simulink model "sampleModel1691"  (R2023a)
settings: Solver=VariableStepAuto  StartTime=0.0  StopTime=10.0  RelTol=1e-3
libraries: hdlsllib x5
settings Model: Creator=user1  LastModifiedBy=user1

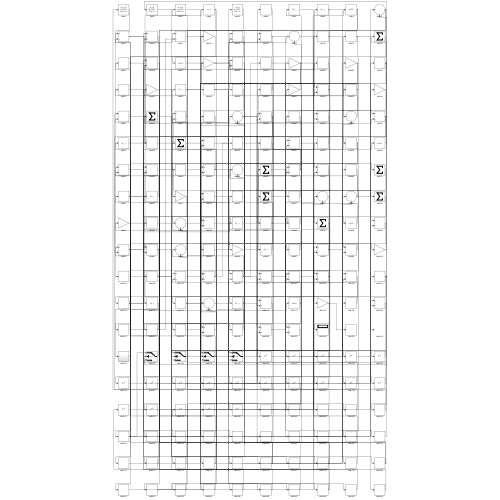
[thumbnail: Simulink's stored preview of the top-level diagram]
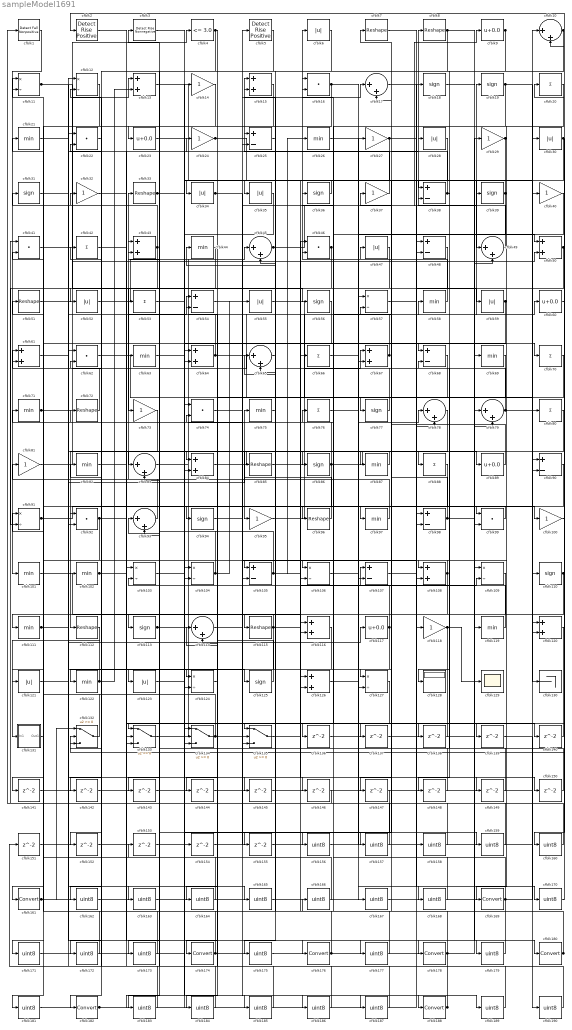
== system sampleModel1691 ==
  cfblk1 : hdlsllib/Logic and Bit Operations/Detect Fall Nonpositive  vinit=0  OutDataTypeStr=boolean
  cfblk{10,17,45,49,65,78..79,83,93,114} (10 alike) : Sum  Inputs=|++
  cfblk{14,24,27,29,32,37,40,73,81,95,100,118} (12 alike) : Gain
  cfblk{21,26,44,58,63,69,71,75,82,87,97,101..102,111,119,122} (16 alike) : MinMax
  cfblk{11..12,57,91,103..104,106,109,124,127} (10 alike) : Product  Inputs=*/  RndMeth=Zero  SaturateOnIntegerOverflow=on
  cfblk{25,38,48,54,68,90,98,105,107} (9 alike) : Sum  Inputs=+-
  cfblk{13,15,43,50,61,64,67,84,108,116,120,126} (12 alike) : Sum
  cfblk{18..19,31,36,39,56,77,86,94,110,113,125} (12 alike) : Signum
  cfblk{7..8,33,51,72,85,96,112,115} (9 alike) : Reshape
  cfblk{9,23,60,89,117} (5 alike) : Bias  Bias=0.0  SaturateOnIntegerOverflow=off
  cfblk{6,28,30,34..35,47,52,55,59,121,123} (11 alike) : Abs  SaturateOnIntegerOverflow=off
  cfblk128 : Display
  cfblk129 : Scope
  cfblk130 : Terminator
  cfblk131 : Subsystem
      settings: LibrarySourceBlock=|
      | hdlsllib/Ports &
      | Subsystems/Subsystem
  cfblk{132..135} (4 alike) : Switch  SaturateOnIntegerOverflow=off  InputSameDT=off
  cfblk{136..155} (20 alike) : Delay  SampleTime=1
  cfblk{156..160,162..168,170..173,175,177,179,181,183..187,189..190} (27 alike) : DataTypeConversion  OutDataTypeStr=uint8  SaturateOnIntegerOverflow=off  RndMeth=Floor
  cfblk{16,22,41,46,62,74,92,99} (8 alike) : DotProduct  OutDataTypeStr=Inherit: Inherit via internal rule
  cfblk{161,169,174,176,178,180,182,188} (8 alike) : DataTypeConversion  SaturateOnIntegerOverflow=off  RndMeth=Floor
  cfblk2 : hdlsllib/Logic and Bit Operations/Detect Rise Positive  vinit=0  OutDataTypeStr=boolean
  cfblk{20,42,53,66,70,76,80,88} (8 alike) : Sum  Inputs=+
  cfblk3 : hdlsllib/Logic and Bit Operations/Detect Rise Nonnegative  vinit=0  OutDataTypeStr=boolean
  cfblk4 : hdlsllib/Logic and Bit Operations/Compare To Constant  relop=<=  const=3.0  OutDataTypeStr=boolean
  cfblk5 : hdlsllib/Logic and Bit Operations/Detect Rise Positive  vinit=0  OutDataTypeStr=boolean
  wires:
  cfblk37/1 -> cfblk15/1
  cfblk36/1 -> cfblk34/1
  cfblk1/1 -> cfblk101/1
  cfblk93/1 -> cfblk33/1
  cfblk133/1 -> cfblk60/1
  cfblk117/1 -> cfblk122/1, cfblk93/1
  cfblk121/1 -> cfblk117/1
  cfblk46/1 -> cfblk73/1, cfblk91/2
  cfblk105/1 -> cfblk43/1, cfblk65/2, cfblk109/2, cfblk26/1
  cfblk113/1 -> cfblk45/1, cfblk187/1
  cfblk51/1 -> cfblk13/1
  cfblk91/1 -> cfblk99/1, cfblk85/1
  cfblk88/1 -> cfblk111/1
  cfblk20/1 -> cfblk169/1
  cfblk95/1 -> cfblk67/1
  cfblk55/1 -> cfblk77/1
  cfblk11/1 -> cfblk56/1, cfblk87/1
  cfblk71/1 -> cfblk4/1, cfblk124/2
  cfblk111/1 -> cfblk54/2, cfblk145/1
  cfblk70/1 -> cfblk106/1
  cfblk45/1 -> cfblk9/1, cfblk149/1
  cfblk100/1 -> cfblk2/1
  cfblk108/1 -> cfblk102/1, cfblk175/1
  cfblk49/1 -> cfblk8/1
  cfblk118/1 -> cfblk129/1, cfblk133/3
  cfblk62/1 -> cfblk130/1
  cfblk48/1 -> cfblk52/1
  cfblk25/1 -> cfblk105/1
  cfblk26/1 -> cfblk48/2
  cfblk134/1 -> cfblk11/2, cfblk140/1
  cfblk79/1 -> cfblk40/1, cfblk25/1
  cfblk68/1 -> cfblk127/1
  cfblk97/1 -> cfblk81/1
  cfblk85/1 -> cfblk19/1
  cfblk99/1 -> cfblk97/1
  cfblk69/1 -> cfblk174/1
  cfblk119/1 -> cfblk107/1
  cfblk86/1 -> cfblk88/1, cfblk94/1, cfblk74/2
  cfblk14/1 -> cfblk161/1
  cfblk78/1 -> cfblk95/1
  cfblk13/1 -> cfblk116/1
  cfblk7/1 -> cfblk50/1
  cfblk89/1 -> cfblk37/1
  cfblk53/1 -> cfblk134/1
  cfblk10/1 -> cfblk115/1, cfblk128/1
  cfblk22/1 -> cfblk182/1
  cfblk96/1 -> cfblk75/1
  cfblk44/1 -> cfblk123/1
  cfblk73/1 -> cfblk112/1
  cfblk19/1 -> cfblk90/1, cfblk86/1
  cfblk43/1 -> cfblk92/1, cfblk31/1
  cfblk112/1 -> cfblk131/1(In1)
  cfblk114/1 -> cfblk188/1
  cfblk58/1 -> cfblk6/1
  cfblk29/1 -> cfblk49/1, cfblk104/2
  cfblk115/1 -> cfblk113/1, cfblk150/1, cfblk173/1
  cfblk94/1 -> cfblk17/1
  cfblk9/1 -> cfblk108/1, cfblk84/2
  cfblk16/1 -> cfblk107/2, cfblk172/1
  cfblk35/1 -> cfblk134/2
  cfblk41/1 -> cfblk50/2
  cfblk50/1 -> cfblk116/2, cfblk135/3
  cfblk65/1 -> cfblk135/1
  cfblk6/1 -> cfblk63/1
  cfblk101/1 -> cfblk126/1
  cfblk23/1 -> cfblk80/1
  cfblk61/1 -> cfblk24/1
  cfblk81/1 -> cfblk58/1
  cfblk72/1 -> cfblk61/1
  cfblk47/1 -> cfblk134/3
  cfblk102/1 -> cfblk28/1, cfblk125/1
  cfblk98/1 -> cfblk79/1, cfblk47/1
  cfblk39/1 -> cfblk35/1, cfblk157/1
  cfblk125/1 -> cfblk71/1
  cfblk106/1 -> cfblk39/1
  cfblk33/1 -> cfblk38/1, cfblk70/1
  cfblk135/1 -> cfblk66/1
  cfblk92/1 -> cfblk152/1, cfblk179/1, cfblk181/1
  cfblk34/1 -> cfblk68/1, cfblk108/2
  cfblk63/1 -> cfblk104/1
  cfblk126/1 -> cfblk78/1
  cfblk59/1 -> cfblk124/1, cfblk92/2
  cfblk109/1 -> cfblk121/1
  cfblk87/1 -> cfblk83/1
  cfblk132/1 -> cfblk91/1
  cfblk42/1 -> cfblk176/1
  cfblk82/1 -> cfblk178/1
  cfblk131/1(Out1) -> cfblk61/2
  cfblk110/1 -> cfblk132/2, cfblk135/2
  cfblk24/1 -> cfblk118/1, cfblk16/2
  cfblk104/1 -> cfblk83/2, cfblk55/1
  cfblk83/1 -> cfblk5/1
  cfblk122/1 -> cfblk11/1, cfblk13/2
  cfblk30/1 -> cfblk64/2, cfblk160/1
  cfblk124/1 -> cfblk54/1
  cfblk84/1 -> cfblk89/1
  cfblk8/1 -> cfblk100/1, cfblk93/2
  cfblk67/1 -> cfblk36/1, cfblk16/1
  cfblk38/1 -> cfblk17/2, cfblk138/1
  cfblk18/1 -> cfblk180/1
  cfblk60/1 -> cfblk10/2
  cfblk52/1 -> cfblk38/2
  cfblk15/1 -> cfblk23/1
  cfblk4/1 -> cfblk84/1, cfblk162/1
  cfblk27/1 -> cfblk59/1, cfblk127/2, cfblk96/1
  cfblk77/1 -> cfblk44/1
  cfblk64/1 -> cfblk120/2, cfblk53/1
  cfblk40/1 -> cfblk136/1
  cfblk136/1 -> cfblk79/2
  cfblk2/1 -> cfblk137/1
  cfblk137/1 -> cfblk49/2
  cfblk138/1 -> cfblk133/2
  cfblk17/1 -> cfblk139/1
  cfblk140/1 -> cfblk133/1
  cfblk56/1 -> cfblk141/1
  cfblk141/1 -> cfblk126/2
  cfblk5/1 -> cfblk142/1
  cfblk142/1 -> cfblk10/1
  cfblk116/1 -> cfblk143/1
  cfblk143/1 -> cfblk106/2
  cfblk90/1 -> cfblk144/1
  cfblk144/1 -> cfblk67/2
  cfblk145/1 -> cfblk120/1
  cfblk74/1 -> cfblk146/1
  cfblk146/1 -> cfblk1/1
  cfblk28/1 -> cfblk147/1
  cfblk80/1 -> cfblk148/1
  cfblk148/1 -> cfblk15/2
  cfblk149/1 -> cfblk43/2
  cfblk150/1 -> cfblk68/2
  cfblk151/1 -> cfblk105/2
  cfblk152/1 -> cfblk25/2
  cfblk153/1 -> cfblk98/2
  cfblk154/1 -> cfblk78/2
  cfblk75/1 -> cfblk155/1
  cfblk155/1 -> cfblk27/1
  cfblk3/1 -> cfblk156/1
  cfblk156/1 -> cfblk30/1
  cfblk157/1 -> cfblk3/1
  cfblk57/1 -> cfblk158/1
  cfblk158/1 -> cfblk41/1
  cfblk123/1 -> cfblk159/1
  cfblk159/1 -> cfblk57/1
  cfblk160/1 -> cfblk57/2
  cfblk161/1 -> cfblk64/1, cfblk109/1, cfblk41/2, cfblk132/1
  cfblk162/1 -> cfblk14/1
  cfblk21/1 -> cfblk163/1
  cfblk163/1 -> cfblk110/1
  cfblk120/1 -> cfblk164/1
  cfblk164/1 -> cfblk21/1
  cfblk32/1 -> cfblk165/1
  cfblk165/1 -> cfblk99/2
  cfblk166/1 -> cfblk32/1
  cfblk76/1 -> cfblk167/1
  cfblk167/1 -> cfblk90/2
  cfblk66/1 -> cfblk168/1
  cfblk168/1 -> cfblk76/1
  cfblk169/1 -> cfblk166/1, cfblk48/1
  cfblk107/1 -> cfblk170/1
  cfblk170/1 -> cfblk20/1
  cfblk12/1 -> cfblk171/1
  cfblk171/1 -> cfblk74/1
  cfblk172/1 -> cfblk12/1
  cfblk173/1 -> cfblk12/2
  cfblk174/1 -> cfblk132/3, cfblk29/1
  cfblk175/1 -> cfblk69/1
  cfblk176/1 -> cfblk153/1, cfblk119/1, cfblk51/1, cfblk72/1
  cfblk31/1 -> cfblk177/1
  cfblk177/1 -> cfblk42/1
  cfblk178/1 -> cfblk151/1, cfblk7/1, cfblk65/1, cfblk45/2
  cfblk179/1 -> cfblk82/1
  cfblk180/1 -> cfblk46/2, cfblk46/1
  cfblk181/1 -> cfblk18/1
  cfblk182/1 -> cfblk154/1, cfblk189/1
  cfblk147/1 -> cfblk183/1
  cfblk183/1 -> cfblk22/1
  cfblk127/1 -> cfblk184/1
  cfblk184/1 -> cfblk22/2
  cfblk103/1 -> cfblk185/1
  cfblk185/1 -> cfblk62/2
  cfblk54/1 -> cfblk186/1
  cfblk186/1 -> cfblk103/1
  cfblk187/1 -> cfblk103/2
  cfblk188/1 -> cfblk98/1, cfblk62/1
  cfblk189/1 -> cfblk114/1
  cfblk139/1 -> cfblk190/1
  cfblk190/1 -> cfblk114/2

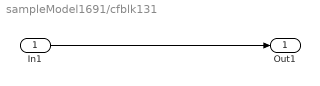
== system sampleModel1691/cfblk131 ==
  In1 : Inport
  Out1 : Outport
  wires:
  In1/1 -> Out1/1
